simulink model "robot"  (Simulink 8.8)
settings: Solver=ode45  StartTime=0.0  StopTime=10  RelTol=1e-3  EnableMultiTasking=on
PreLoadFcn:
  | Factory
InitFcn:
  | Factory
values from neighbouring files (symbols this model uses):
  Amp1d = [R1*R2*C2 R1]    [Robot.m]
  Amp1n = [R1*R2*(C1+C2) R1+R2]    [Robot.m]
  Amp2d = [R1*R2*C2 R1]    [Robot.m]
  Amp2n = [R1*R2*(C1+C2) R1+R2]    [Robot.m]
  AmpSat1 = VSS    [Robot.m]
  AmpSat2 = VSS    [Robot.m]
  BackEMF1 = 1/ME    [Robot.m]
  BackEMF2 = 1/ME    [Robot.m]
  Elec1d = [ML MR]    [Robot.m]
  Elec2d = [ML MR]    [Robot.m]
  FB0 = 1    [Robot.m]
  FB1 = 1    [Robot.m]
  FB2 = 1    [Robot.m]
  Gear1 = 1/GR1    [Robot.m]
  Gear2 = 1/GR2    [Robot.m]
  Grav = G*M1*L1/2 + G*(MM + GM2)*L1    [Robot.m]
  JntMax0 = QU0    [Robot.m]
  JntMax1 = QU1    [Robot.m]
  JntMax2 = QU2    [Robot.m]
  JntMin0 = QL0    [Robot.m]
  JntMin1 = QL1    [Robot.m]
  JntMin2 = QL2    [Robot.m]
  Mech0d = [M0 B0]    [Robot.m]
  Mech0n = pi*(ID0/2)^2    [Robot.m]
  Mech1d = [MJ+GJ1+((M1*(L1/2)^2)+MM*L1^2+GM2*L1^2)/(GR1^2) MB+GB1]    [Robot.m]
  Mech2d = [MJ+GJ2 MB+GB2]    [Robot.m]
  Pump0d = [PT0 1]    [Robot.m]
  Pump0n = PK0    [Robot.m]
  Pump0sat = PM0    [Robot.m]
  TConst1 = MT    [Robot.m]
  TConst2 = MT    [Robot.m]
undefined symbols (not defined in the file or in its folder): Elec1n, Elec2n, GR1, GR2, Mech1n, Mech2n
libraries: simulink x3, vrlib x1
settings Model: LogicAnalyzerSignalOrdering=f835d39d-8e1e-492a-b14b-cd398f1bf1ae  Creator=Leos  LastModifiedBy=Graham
settings DataIOCC: LimitDataPoints=off
settings OptimizationCC: ExpressionDepthLimit=2147483647
settings DebuggingCC: SolverPrmCheckMsg=warning
settings ConfigComp: CovSFcnEnable=off

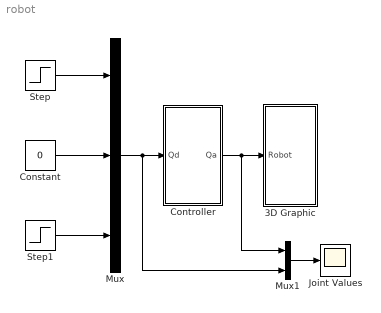
== system robot ==
  3D Graphic : Subsystem
  Constant : Constant  Value=0
  Controller : Subsystem
  Joint Values : Scope
  Mux : Mux  Inputs=3
  Mux1 : Mux  Inputs=2
  Step : Step  SampleTime=0
  Step1 : Step  Time=.5  Before=pi/2  After=0  SampleTime=0
  wires:
  Mux/1 -> Controller/1(Qd), Mux1/2
  Controller/1(Qa) -> Mux1/1, 3D Graphic/1(Robot)
  Mux1/1 -> Joint Values/1
  Constant/1 -> Mux/2
  Step/1 -> Mux/1
  Step1/1 -> Mux/3

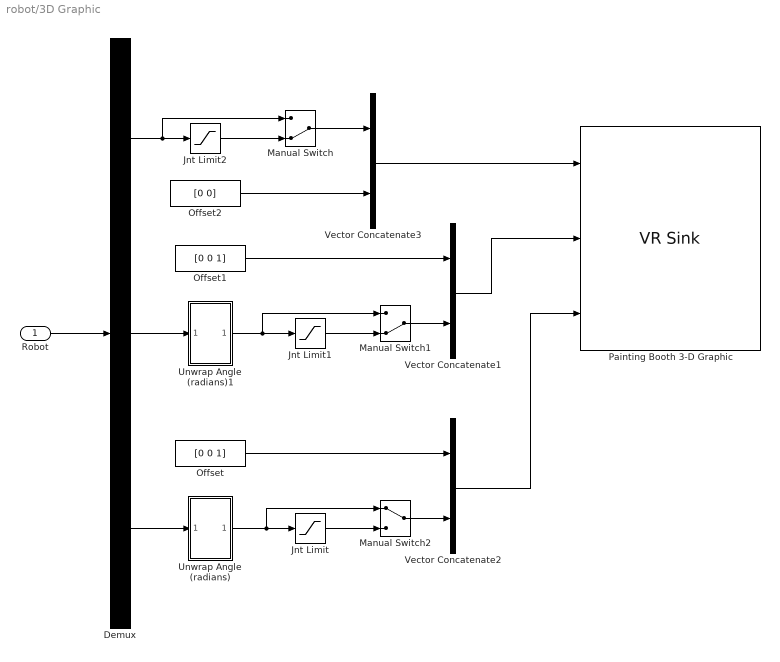
== system robot/3D Graphic ==
  Robot : Inport
  Demux : Demux  Outputs=3
  Jnt Limit : Saturate  UpperLimit=4*pi/5  LowerLimit=-4*pi/5
  Jnt Limit1 : Saturate  UpperLimit=pi/2  LowerLimit=-pi
  Jnt Limit2 : Saturate  UpperLimit=4.5  LowerLimit=-.5
  Manual Switch : ManualSwitch  CurrentSetting=0
  Manual Switch1 : ManualSwitch  CurrentSetting=0
  Manual Switch2 : ManualSwitch
  Offset : Constant  Value=[0 0 1]
  Offset1 : Constant  Value=[0 0 1]
  Offset2 : Constant  Value=[0 0]
  Painting Booth 3-D Graphic : vrlib/VR Sink  InstantiateOnLoad=on  SampleTime=-1  ViewEnable=on  RemoteChange=off  RemoteView=off  FieldsWritten=Q0.translation.3.1.1.double#Q1.rotation.4.1.1.double#Q2.rotation.4.1.1.double  WorldFileName=ROBOT.WRL  AutoView=on  VideoDimensions=[]  AllowVariableSize=off  FigureProperties="{'Position', 'Name', 'Viewpoint', 'CameraBound', 'CameraDirection', 'CameraPosition', 'CameraUpVector', 'ZoomFactor', 'Antialiasing', 'Headlight', 'Lighting', 'NavPanel', 'Sound', 'StatusBar', 'Stereo3D', 'Stereo3DCameraOffset', 'Stereo3DHIT', 'ToolBar', 'Textures', 'Transparency', 'Triad', 'Wireframe', 'NavZones', 'NavMode', 'NavSpeed', 'CaptureFileFormat', 'CaptureFileName', 'Record2DCompressMethod', 'Record2DCompressQuality', 'Record2D', 'Record2DFileName', 'Record2DFPS'; [5.0000000000000000e+00   9.2000000000000000e+01   5.7600000000000000e+02   3.5000000000000000e+02], '', '_untitled_1', 'on', [0.0000000000000000e+00   0.0000000000000000e+00  -1.0000000000000000e+00], [0.0000000000000000e+00   0.0000000000000000e+00   0.0000000000000000e+00], [0.0000000000000000e+00   1.0000000000000000e+00   0.0000000000000000e+00], [1.0000000000000000e+00], 'on', 'off', 'on', 'halfbar', 'on', 'on', 'off', [1.0000000149011612e-01], [0.0000000000000000e+00], 'on', 'on', 'on', 'none', 'off', 'off', 'walk', 'normal', 'tif', '%f_anim_%n.tif', 'auto', [7.5000000000000000e+01], 'off', '%f_anim_%n.avi', 'auto'}"
  Unwrap Angle (radians) : Subsystem
  Unwrap Angle (radians)1 : Subsystem
  Vector Concatenate1 : Concatenate
  Vector Concatenate2 : Concatenate
  Vector Concatenate3 : Concatenate
  wires:
  Unwrap Angle (radians)/1(Out1) -> Manual Switch2/1, Jnt Limit/1
  Offset/1 -> Vector Concatenate2/1
  Unwrap Angle (radians)1/1(Out1) -> Manual Switch1/1, Jnt Limit1/1
  Offset1/1 -> Vector Concatenate1/1
  Offset2/1 -> Vector Concatenate3/2
  Robot/1 -> Demux/1
  Demux/1 -> Manual Switch/1, Jnt Limit2/1
  Demux/2 -> Unwrap Angle (radians)1/1(In1)
  Demux/3 -> Unwrap Angle (radians)/1(In1)
  Vector Concatenate3/1 -> Painting Booth 3-D Graphic/1
  Vector Concatenate1/1 -> Painting Booth 3-D Graphic/2
  Vector Concatenate2/1 -> Painting Booth 3-D Graphic/3
  Manual Switch/1 -> Vector Concatenate3/1
  Jnt Limit2/1 -> Manual Switch/2
  Manual Switch1/1 -> Vector Concatenate1/2
  Jnt Limit1/1 -> Manual Switch1/2
  Jnt Limit/1 -> Manual Switch2/2
  Manual Switch2/1 -> Vector Concatenate2/2

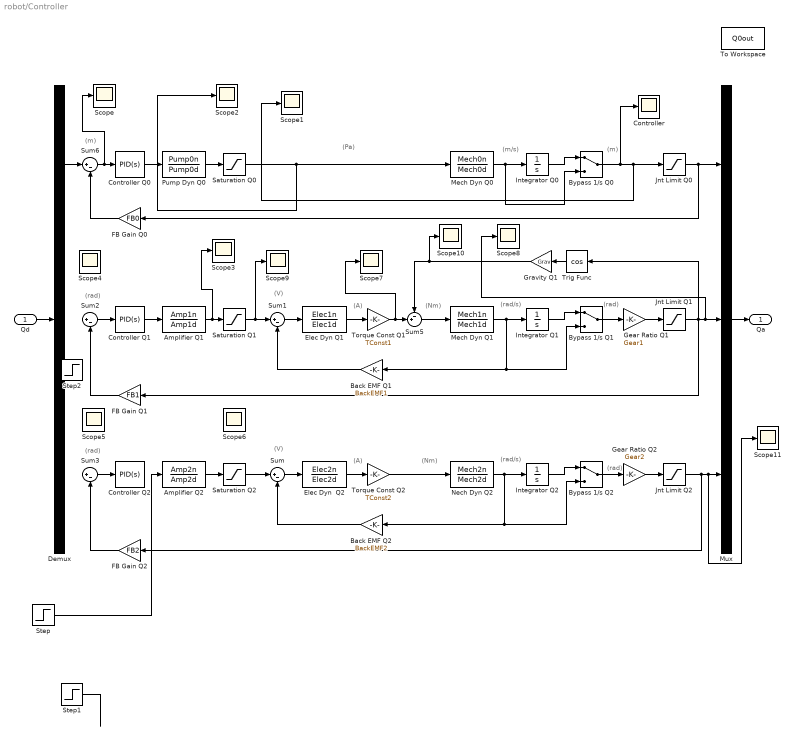
== system robot/Controller ==
  note: (rad)
  note: (V)
  note: (rad/s)
  note: (rad)
  note: (A)
  note: (Nm)
  note: (rad)
  note: (V)
  note: (rad/s)
  note: (rad)
  note: (A)
  note: (Nm)
  note: (m)
  note: (m)
  note: (Pa)
  note: (m/s)
  Qd : Inport
  Amplifier Q1 : TransferFcn  Numerator=Amp1n  Denominator=Amp1d
  Amplifier Q2 : TransferFcn  Numerator=Amp2n  Denominator=Amp2d
  Back EMF Q1 : Gain  Gain=BackEMF1
  Back EMF Q2 : Gain  Gain=BackEMF2
  Bypass 1/s Q0 : ManualSwitch
  Bypass 1/s Q1 : ManualSwitch
  Bypass 1/s Q2 : ManualSwitch
  Controller : Scope
  Controller Q0 : simulink/Continuous/PID Controller  Controller=PID  TimeDomain=Continuous-time  SampleTime=-1  IntegratorMethod=Forward Euler  FilterMethod=Forward Euler  Form=Parallel  UseFilter=on  ControllerParametersSource=internal  P=8.63538835045854e-06  I=1.50501796285065e-06  D=7.57196247349536e-06  N=7.46661935266962  InitialConditionSource=internal  InitialConditionForIntegrator=0  InitialConditionForFilter=0  ExternalReset=none  LimitOutput=off  UpperSaturationLimit=inf  LowerSaturationLimit=-inf  LinearizeAsGain=on  AntiWindupMode=none  Kb=1  TrackingMode=off  Kt=1  PParamMin=[]  PParamMax=[]  IParamMin=[]  IParamMax=[]  DParamMin=[]  DParamMax=[]  NParamMin=[]  NParamMax=[]  KbParamMin=[]  KbParamMax=[]  KtParamMin=[]  KtParamMax=[]  POutMin=[]  POutMax=[]  IOutMin=[]  IOutMax=[]  DOutMin=[]  DOutMax=[]  NOutMin=[]  NOutMax=[]  KbOutMin=[]  KbOutMax=[]  KtOutMin=[]  KtOutMax=[]  IntegratorOutMin=[]  IntegratorOutMax=[]  FilterOutMin=[]  FilterOutMax=[]  SumOutMin=[]  SumOutMax=[]  SumI1OutMin=[]  SumI1OutMax=[]  SumI2OutMin=[]  SumI2OutMax=[]  SumI3OutMin=[]  SumI3OutMax=[]  SumDOutMin=[]  SumDOutMax=[]  SaturationOutMin=[]  SaturationOutMax=[]  IntegratorContinuousStateAttributes=''  IntegratorStateMustResolveToSignalObject=off  IntegratorRTWStateStorageClass=Auto  FilterContinuousStateAttributes=''  FilterStateMustResolveToSignalObject=off  FilterRTWStateStorageClass=Auto  DifferentiatorICPrevScaledInput=0  DifferentiatorOutMin=[]  DifferentiatorOutMax=[]
  Controller Q1 : simulink/Continuous/PID Controller  Controller=PID  TimeDomain=Continuous-time  SampleTime=-1  IntegratorMethod=Forward Euler  FilterMethod=Forward Euler  Form=Parallel  UseFilter=on  ControllerParametersSource=internal  P=3.24017627577691  I=4.01004122358437  D=-0.137704932094223  N=1.91327738186974  InitialConditionSource=internal  InitialConditionForIntegrator=0  InitialConditionForFilter=0  ExternalReset=none  LimitOutput=off  UpperSaturationLimit=inf  LowerSaturationLimit=-inf  LinearizeAsGain=on  AntiWindupMode=none  Kb=1  TrackingMode=off  Kt=1  PParamMin=[]  PParamMax=[]  IParamMin=[]  IParamMax=[]  DParamMin=[]  DParamMax=[]  NParamMin=[]  NParamMax=[]  KbParamMin=[]  KbParamMax=[]  KtParamMin=[]  KtParamMax=[]  POutMin=[]  POutMax=[]  IOutMin=[]  IOutMax=[]  DOutMin=[]  DOutMax=[]  NOutMin=[]  NOutMax=[]  KbOutMin=[]  KbOutMax=[]  KtOutMin=[]  KtOutMax=[]  IntegratorOutMin=[]  IntegratorOutMax=[]  FilterOutMin=[]  FilterOutMax=[]  SumOutMin=[]  SumOutMax=[]  SumI1OutMin=[]  SumI1OutMax=[]  SumI2OutMin=[]  SumI2OutMax=[]  SumI3OutMin=[]  SumI3OutMax=[]  SumDOutMin=[]  SumDOutMax=[]  SaturationOutMin=[]  SaturationOutMax=[]  IntegratorContinuousStateAttributes=''  IntegratorStateMustResolveToSignalObject=off  IntegratorRTWStateStorageClass=Auto  FilterContinuousStateAttributes=''  FilterStateMustResolveToSignalObject=off  FilterRTWStateStorageClass=Auto  DifferentiatorICPrevScaledInput=0  DifferentiatorOutMin=[]  DifferentiatorOutMax=[]
  Controller Q2 : simulink/Continuous/PID Controller  Controller=PID  TimeDomain=Continuous-time  SampleTime=-1  IntegratorMethod=Forward Euler  FilterMethod=Forward Euler  Form=Parallel  UseFilter=on  ControllerParametersSource=internal  P=27.5316312668747  I=187.405964313373  D=-0.0979825076020959  N=188.62638742826  InitialConditionSource=internal  InitialConditionForIntegrator=0  InitialConditionForFilter=0  ExternalReset=none  LimitOutput=off  UpperSaturationLimit=inf  LowerSaturationLimit=-inf  LinearizeAsGain=on  AntiWindupMode=none  Kb=1  TrackingMode=off  Kt=1  PParamMin=[]  PParamMax=[]  IParamMin=[]  IParamMax=[]  DParamMin=[]  DParamMax=[]  NParamMin=[]  NParamMax=[]  KbParamMin=[]  KbParamMax=[]  KtParamMin=[]  KtParamMax=[]  POutMin=[]  POutMax=[]  IOutMin=[]  IOutMax=[]  DOutMin=[]  DOutMax=[]  NOutMin=[]  NOutMax=[]  KbOutMin=[]  KbOutMax=[]  KtOutMin=[]  KtOutMax=[]  IntegratorOutMin=[]  IntegratorOutMax=[]  FilterOutMin=[]  FilterOutMax=[]  SumOutMin=[]  SumOutMax=[]  SumI1OutMin=[]  SumI1OutMax=[]  SumI2OutMin=[]  SumI2OutMax=[]  SumI3OutMin=[]  SumI3OutMax=[]  SumDOutMin=[]  SumDOutMax=[]  SaturationOutMin=[]  SaturationOutMax=[]  IntegratorContinuousStateAttributes=''  IntegratorStateMustResolveToSignalObject=off  IntegratorRTWStateStorageClass=Auto  FilterContinuousStateAttributes=''  FilterStateMustResolveToSignalObject=off  FilterRTWStateStorageClass=Auto  DifferentiatorICPrevScaledInput=0  DifferentiatorOutMin=[]  DifferentiatorOutMax=[]
  Demux : Demux  Outputs=3
  Elec Dyn Q1 : TransferFcn  Numerator=Elec1n  Denominator=Elec1d
  Elec Dyn  Q2 : TransferFcn  Numerator=Elec2n  Denominator=Elec2d
  FB Gain Q0 : Gain  Gain=FB0
  FB Gain Q1 : Gain  Gain=FB1
  FB Gain Q2 : Gain  Gain=FB2
  Gear Ratio Q1 : Gain  Gain=Gear1
  Gear Ratio Q2 : Gain  Gain=Gear2
  Gravity Q1 : Gain  Gain=Grav
  Integrator Q0 : Integrator
  Integrator Q1 : Integrator  InitialCondition=-pi/2*GR1
  Integrator Q2 : Integrator  InitialCondition=pi/2*GR2
  Jnt Limit Q0 : Saturate  UpperLimit=JntMax0  LowerLimit=JntMin0
  Jnt Limit Q1 : Saturate  UpperLimit=JntMax1  LowerLimit=JntMin1
  Jnt Limit Q2 : Saturate  UpperLimit=JntMax2  LowerLimit=JntMin2
  Mech Dyn Q0 : TransferFcn  Numerator=Mech0n  Denominator=Mech0d
  Mech Dyn Q1 : TransferFcn  Numerator=Mech1n  Denominator=Mech1d
  Mux : Mux  Inputs=3
  Nech Dyn Q2 : TransferFcn  Numerator=Mech2n  Denominator=Mech2d
  Pump Dyn Q0 : TransferFcn  Numerator=Pump0n  Denominator=Pump0d
  Saturation Q0 : Saturate  UpperLimit=Pump0sat  LowerLimit=-Pump0sat
  Saturation Q1 : Saturate  UpperLimit=AmpSat1  LowerLimit=-AmpSat1
  Saturation Q2 : Saturate  UpperLimit=AmpSat2  LowerLimit=-AmpSat2
  Scope{,1..11} (12 alike) : Scope
  Step : Step  Time=0  SampleTime=0
  Step1 : Step  SampleTime=0
  Step2 : Step  SampleTime=0
  Sum{,1..3,6} (5 alike) : Sum  Inputs=|+-
  Sum5 : Sum  Inputs=-+|
  To Workspace : ToWorkspace  VariableName=Q0out  SaveFormat=Timeseries  SampleTime=-1
  Torque Const Q1 : Gain  Gain=TConst1
  Torque Const Q2 : Gain  Gain=TConst2
  Trig Func : Trigonometry  Operator=cos
  Qa : Outport
  wires:
  Qd/1 -> Demux/1
  Mux/1 -> Qa/1
  Sum/1 -> Elec Dyn  Q2/1
  Sum3/1 -> Controller Q2/1
  Amplifier Q2/1 -> Saturation Q2/1
  Saturation Q2/1 -> Sum/1
  Back EMF Q2/1 -> Sum/2
  Torque Const Q2/1 -> Nech Dyn Q2/1
  FB Gain Q2/1 -> Sum3/2
  Nech Dyn Q2/1 -> Integrator Q2/1, Bypass 1/s Q2/2, Back EMF Q2/1
  Sum1/1 -> Elec Dyn Q1/1
  Sum2/1 -> Controller Q1/1
  Elec Dyn Q1/1 -> Torque Const Q1/1
  Amplifier Q1/1 -> Scope3/1, Saturation Q1/1
  Saturation Q1/1 -> Scope9/1, Sum1/1
  Back EMF Q1/1 -> Sum1/2
  Mech Dyn Q1/1 -> Integrator Q1/1, Bypass 1/s Q1/2, Back EMF Q1/1
  Torque Const Q1/1 -> Scope7/1, Sum5/2
  Sum5/1 -> Mech Dyn Q1/1
  Saturation Q0/1 -> Scope2/1, Mech Dyn Q0/1
  Sum6/1 -> Scope/1, Controller Q0/1
  Pump Dyn Q0/1 -> Saturation Q0/1
  FB Gain Q0/1 -> Sum6/2
  Trig Func/1 -> Gravity Q1/1
  Gravity Q1/1 -> Scope10/1, Sum5/1
  Bypass 1/s Q2/1 -> Gear Ratio Q2/1
  Bypass 1/s Q1/1 -> Gear Ratio Q1/1
  Integrator Q1/1 -> Bypass 1/s Q1/1
  Integrator Q2/1 -> Bypass 1/s Q2/1
  Integrator Q0/1 -> Bypass 1/s Q0/1
  Mech Dyn Q0/1 -> Bypass 1/s Q0/2, Integrator Q0/1
  Jnt Limit Q0/1 -> Mux/1, FB Gain Q0/1
  Gear Ratio Q1/1 -> Jnt Limit Q1/1
  Jnt Limit Q1/1 -> FB Gain Q1/1, Scope8/1, Mux/2, Trig Func/1
  Gear Ratio Q2/1 -> Jnt Limit Q2/1
  Jnt Limit Q2/1 -> FB Gain Q2/1, Scope11/1, Mux/3
  Elec Dyn  Q2/1 -> Torque Const Q2/1
  Bypass 1/s Q0/1 -> Controller/1, Scope1/1, Jnt Limit Q0/1
  FB Gain Q1/1 -> Sum2/2
  Demux/1 -> Sum6/1
  Controller Q1/1 -> Amplifier Q1/1
  Controller Q0/1 -> Pump Dyn Q0/1
  Step1/1 -> ?
  Step/1 -> Amplifier Q2/1

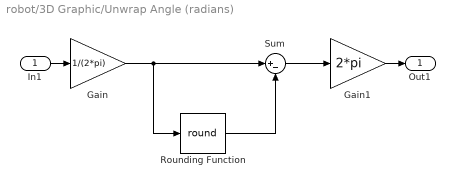
== system robot/3D Graphic/Unwrap Angle (radians) ==
  In1 : Inport
  Gain : Gain  Gain=1/(2*pi)
  Gain1 : Gain  Gain=2*pi
  Rounding Function : Rounding  Operator=round
  Sum : Sum  Inputs=|+-
  Out1 : Outport
  wires:
  Gain/1 -> Rounding Function/1, Sum/1
  Rounding Function/1 -> Sum/2
  Sum/1 -> Gain1/1
  In1/1 -> Gain/1
  Gain1/1 -> Out1/1

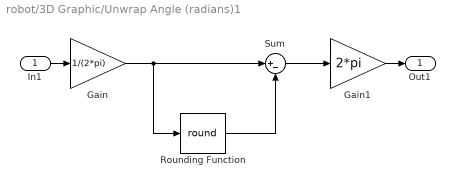
== system robot/3D Graphic/Unwrap Angle (radians)1 ==
  In1 : Inport
  Gain : Gain  Gain=1/(2*pi)
  Gain1 : Gain  Gain=2*pi
  Rounding Function : Rounding  Operator=round
  Sum : Sum  Inputs=|+-
  Out1 : Outport
  wires:
  Gain/1 -> Rounding Function/1, Sum/1
  Rounding Function/1 -> Sum/2
  Sum/1 -> Gain1/1
  In1/1 -> Gain/1
  Gain1/1 -> Out1/1
